simulink library "actuator_processing"  (R2016b)
settings: Solver=VariableStepAuto  StartTime=0.0  StopTime=10.0  RelTol=1e-3
settings Model: Creator=taylorreynolds  LastModifiedBy=Taylor

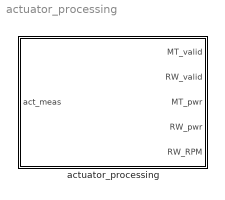
== system actuator_processing ==
  actuator_processing : Subsystem

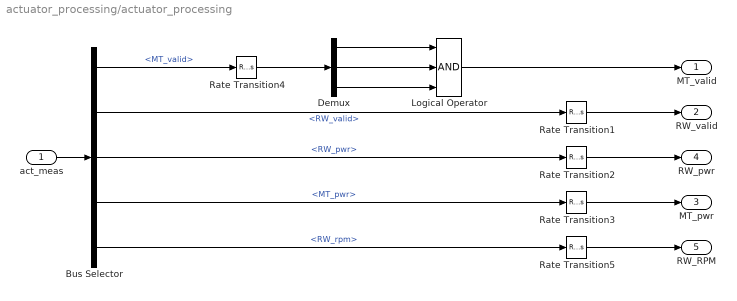
== system actuator_processing/actuator_processing ==
  act_meas : Inport
  Bus Selector : BusSelector  OutputSignals=MT_valid,RW_valid,RW_pwr,MT_pwr,RW_rpm
  Demux : Demux  Outputs=[1 1 1]
  Logical Operator : Logic  Inputs=3  AllPortsSameDT=off  OutDataTypeStr=boolean
  Rate Transition{1..5} (5 alike) : RateTransition  OutPortSampleTime=fsw_params.sample_time_s
  MT_valid : Outport
  RW_valid : Outport  Port=2
  MT_pwr : Outport  Port=3
  RW_pwr : Outport  Port=4
  RW_RPM : Outport  Port=5
  wires:
  Bus Selector/5 -> Rate Transition5/1  "<RW_rpm>"
  Bus Selector/4 -> Rate Transition3/1  "<MT_pwr>"
  Bus Selector/2 -> Rate Transition1/1  "<RW_valid>"
  Bus Selector/1 -> Rate Transition4/1  "<MT_valid>"
  act_meas/1 -> Bus Selector/1
  Rate Transition4/1 -> Demux/1
  Rate Transition1/1 -> RW_valid/1
  Rate Transition2/1 -> RW_pwr/1
  Bus Selector/3 -> Rate Transition2/1  "<RW_pwr>"
  Rate Transition3/1 -> MT_pwr/1
  Rate Transition5/1 -> RW_RPM/1
  Demux/2 -> Logical Operator/2
  Demux/1 -> Logical Operator/1
  Demux/3 -> Logical Operator/3
  Logical Operator/1 -> MT_valid/1
